simulink model "drivingscenarioslx"  (R2020b)
settings: Solver=FixedStepDiscrete  StartTime=0.0  StopTime=20  RelTol=1e-3
model workspace (MAT data in the model file):
  firstWarning = 1
  originalScenarioChecksum = '1C4B111A82F1CB0582BAAC63DE483F4C'
values from neighbouring files (symbols this model uses):
  C = Cc    [LateralDynamicsDT.m]
libraries: drivingscenarioandsensors x2, simulink_extras x1
settings Model: Creator=chnwa  LastModifiedBy=chnwa

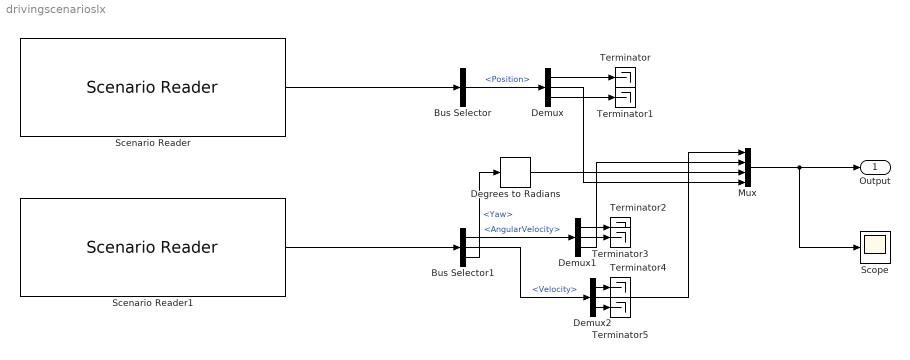
== system drivingscenarioslx ==
  Bus Selector : BusSelector  OutputSignals=Actors.Position
  Bus Selector1 : BusSelector  OutputSignals=Actors.AngularVelocity,Actors.Velocity,Actors.Yaw
  Degrees to Radians : simulink_extras/Transformations/Degrees to Radians
  Demux : Demux  Outputs=3
  Demux1 : Demux  Outputs=3
  Demux2 : Demux  Outputs=3
  Mux : Mux
  Scenario Reader : drivingscenarioandsensors/Scenario Reader  ScenarioSource=From file  ScenarioFileName=C:\Users\Public\Documents\CarSim2017.1_Data\Extensions\Simulink\drivingscenario.mat  ScenarioVariableName=scenario  OutputCoordinateSystem=World coordinates  EgoVehicleSource=Scenario  EgoVehicleActorID=1  OrientVehiclesOnRoad=off  OutputEgoVehiclePose=off  SampleTime=0.1  LaneBoundaryOutput=None  LaneBoundaryDistance=0:0.5:9.5  LaneBoundaryLocation=Center of lane markings  BusNameSource=Auto  BusName=BusActors  BusName2Source=Auto  BusName2=BusLaneBoundaries  BusName3Source=Auto  BusName3=BusEgoActor  ShowCoordinateLabels=on  SimulateUsing=Interpreted execution
  Scenario Reader1 : drivingscenarioandsensors/Scenario Reader  ScenarioSource=From file  ScenarioFileName=C:\Users\Public\Documents\CarSim2017.1_Data\Extensions\Simulink\drivingscenario.mat  ScenarioVariableName=scenario  OutputCoordinateSystem=Vehicle coordinates  EgoVehicleSource=Scenario  EgoVehicleActorID=1  OrientVehiclesOnRoad=off  OutputEgoVehiclePose=off  SampleTime=0.1  LaneBoundaryOutput=None  LaneBoundaryDistance=0:0.5:9.5  LaneBoundaryLocation=Center of lane markings  BusNameSource=Auto  BusName=BusActors  BusName2Source=Auto  BusName2=BusLaneBoundaries  BusName3Source=Auto  BusName3=BusEgoActor  ShowCoordinateLabels=on  SimulateUsing=Interpreted execution
  Scope : Scope
  Terminator{,1..5} (6 alike) : Terminator
  Output : Outport
  wires:
  Bus Selector1/1 -> Demux1/1  "<AngularVelocity>"
  Mux/1 -> Output/1, Scope/1
  Demux/2 -> Mux/4
  Demux/1 -> Terminator/1
  Demux1/2 -> Terminator3/1
  Bus Selector/1 -> Demux/1  "<Position>"
  Demux1/1 -> Terminator2/1
  Demux2/3 -> Terminator5/1
  Scenario Reader1/1 -> Bus Selector1/1
  Demux1/3 -> Mux/2
  Demux2/1 -> Terminator4/1
  Demux/3 -> Terminator1/1
  Demux2/2 -> Mux/1
  Bus Selector1/3 -> Degrees to Radians/1  "<Yaw>"
  Bus Selector1/2 -> Demux2/1  "<Velocity>"
  Scenario Reader/1 -> Bus Selector/1
  Degrees to Radians/1 -> Mux/3
